simulink model "case8"  (R2024b)
settings: Solver=FixedStepAuto  StartTime=0  StopTime=1  FixedStep=1e-7  RelTol=1e-3
values from neighbouring files (symbols this model uses):
  SG_D_1_D = 0.01056    [IEEE9_case_parameters.m]    (also in case1_parameters.m; case2_parameters.m; case3_parameters.m; case4_parameters.m)
  SG_D_1_EnableSaturation = 0    [IEEE9_case_parameters.m]    (also in case1_parameters.m; case2_parameters.m; case3_parameters.m; case4_parameters.m)
  SG_D_1_f0 = 60    [IEEE9_case_parameters.m]    (also in case1_parameters.m; case2_parameters.m; case3_parameters.m; case4_parameters.m)
  SG_D_1_H = 7.5    [IEEE9_case_parameters.m]    (also in case1_parameters.m; case2_parameters.m; case3_parameters.m; case4_parameters.m)
  SG_D_1_K_A = 20    [IEEE9_case_parameters.m]    (also in case1_parameters.m; case2_parameters.m; case3_parameters.m; case4_parameters.m)
  SG_D_1_K_E = 1.000000e+1    (= 10)    [IEEE9_case_parameters.m]    (also in case1_parameters.m; case2_parameters.m; case3_parameters.m; case4_parameters.m)
  SG_D_1_K_F = 2.363    [IEEE9_case_parameters.m]    (also in case1_parameters.m; case2_parameters.m; case3_parameters.m; case4_parameters.m)
  SG_D_1_K_s = 0.5    [IEEE9_case_parameters.m]    (also in case1_parameters.m = 5; case2_parameters.m = 5; case3_parameters.m = 5; case4_parameters.m = 5)
  SG_D_1_R_a = 0.001088    [IEEE9_case_parameters.m]    (also in case1_parameters.m; case2_parameters.m; case3_parameters.m; case4_parameters.m)
  SG_D_1_S_A = 1    [IEEE9_case_parameters.m]    (also in case1_parameters.m; case2_parameters.m; case3_parameters.m; case4_parameters.m)
  SG_D_1_S_B = 0.103    [IEEE9_case_parameters.m]    (also in case1_parameters.m; case2_parameters.m; case3_parameters.m; case4_parameters.m)
  SG_D_1_S_N = 10.659857    [IEEE9_case_parameters.m]    (also in case1_parameters.m; case2_parameters.m; case3_parameters.m; case4_parameters.m)
  SG_D_1_SpeedPara = 200    [IEEE9_case_parameters.m]    (also in case1_parameters.m; case2_parameters.m; case3_parameters.m; case4_parameters.m)
  SG_D_1_T_0 = 0.720173    [IEEE9_case_parameters.m]    (also in case1_parameters.m = 0.755522; case2_parameters.m = 0.808931; case3_parameters.m = 0.869402; case4_parameters.m = 0.729316)
  SG_D_1_T_1 = 0.3    [IEEE9_case_parameters.m]    (also in case1_parameters.m; case2_parameters.m; case3_parameters.m; case4_parameters.m)
  SG_D_1_T_2 = 0.05    [IEEE9_case_parameters.m]    (also in case1_parameters.m; case2_parameters.m; case3_parameters.m; case4_parameters.m)
  SG_D_1_T_3 = 0.02    [IEEE9_case_parameters.m]    (also in case1_parameters.m; case2_parameters.m; case3_parameters.m; case4_parameters.m)
  SG_D_1_T_4 = 0.005    [IEEE9_case_parameters.m]    (also in case1_parameters.m; case2_parameters.m; case3_parameters.m; case4_parameters.m)
  SG_D_1_T_A = 0.02    [IEEE9_case_parameters.m]    (also in case1_parameters.m; case2_parameters.m; case3_parameters.m; case4_parameters.m)
  SG_D_1_T_dd = 8.000000e+0    (= 8)    [IEEE9_case_parameters.m]    (also in case1_parameters.m; case2_parameters.m; case3_parameters.m; case4_parameters.m)
  SG_D_1_T_ddd = 0.04    [IEEE9_case_parameters.m]    (also in case1_parameters.m; case2_parameters.m; case3_parameters.m; case4_parameters.m)
  SG_D_1_T_E = 0.314    [IEEE9_case_parameters.m]    (also in case1_parameters.m; case2_parameters.m; case3_parameters.m; case4_parameters.m)
  SG_D_1_T_F = 0.35    [IEEE9_case_parameters.m]    (also in case1_parameters.m; case2_parameters.m; case3_parameters.m; case4_parameters.m)
  SG_D_1_T_qd = 0.8    [IEEE9_case_parameters.m]    (also in case1_parameters.m; case2_parameters.m; case3_parameters.m; case4_parameters.m)
  SG_D_1_T_qdd = 0.02    [IEEE9_case_parameters.m]    (also in case1_parameters.m; case2_parameters.m; case3_parameters.m; case4_parameters.m)
  SG_D_1_T_speed = 0.1    [IEEE9_case_parameters.m]    (also in case1_parameters.m = 200; case2_parameters.m = 200; case3_parameters.m = 200; case4_parameters.m = 200)
  SG_D_1_T_w = 0.5    [IEEE9_case_parameters.m]    (also in case1_parameters.m; case2_parameters.m; case3_parameters.m; case4_parameters.m)
  SG_D_1_V_ref = 1.990276    [IEEE9_case_parameters.m]    (also in case1_parameters.m = 2.042296; case2_parameters.m = 2.051388; case3_parameters.m = 2.089584; case4_parameters.m = 2.01845)
  SG_D_1_w_ref = 376.991118    [IEEE9_case_parameters.m]    (also in case1_parameters.m; case2_parameters.m; case3_parameters.m; case4_parameters.m)
  SG_D_1_wb = 6.000000e+1    (= 60)    [IEEE9_case_parameters.m]    (also in case1_parameters.m; case2_parameters.m; case3_parameters.m; case4_parameters.m)
  SG_D_1_x_d = 1.9    [IEEE9_case_parameters.m]    (also in case1_parameters.m; case2_parameters.m; case3_parameters.m; case4_parameters.m)
  SG_D_1_x_dd = 0.302    [IEEE9_case_parameters.m]    (also in case1_parameters.m; case2_parameters.m; case3_parameters.m; case4_parameters.m)
  SG_D_1_x_ddd = 0.204    [IEEE9_case_parameters.m]    (also in case1_parameters.m; case2_parameters.m; case3_parameters.m; case4_parameters.m)
  SG_D_1_x_l = 0.05    [IEEE9_case_parameters.m]    (also in case1_parameters.m; case2_parameters.m; case3_parameters.m; case4_parameters.m)
  SG_D_1_x_q = 1.3    [IEEE9_case_parameters.m]    (also in case1_parameters.m; case2_parameters.m; case3_parameters.m; case4_parameters.m)
  SG_D_1_x_qd = 0.5    [IEEE9_case_parameters.m]    (also in case1_parameters.m; case2_parameters.m; case3_parameters.m; case4_parameters.m)
  SG_D_1_x_qdd = 0.3    [IEEE9_case_parameters.m]    (also in case1_parameters.m; case2_parameters.m; case3_parameters.m; case4_parameters.m)
  SG_D_2_D = 0.02    [IEEE9_case_parameters.m]    (also in case1_parameters.m; case2_parameters.m; case3_parameters.m; case4_parameters.m)
  SG_D_2_EnableSaturation = 0    [IEEE9_case_parameters.m]    (also in case1_parameters.m; case2_parameters.m; case3_parameters.m; case4_parameters.m)
  SG_D_2_f0 = 60    [IEEE9_case_parameters.m]    (also in case1_parameters.m; case2_parameters.m; case3_parameters.m; case4_parameters.m)
  SG_D_2_H = 8.000000e+0    (= 8)    [IEEE9_case_parameters.m]    (also in case1_parameters.m; case2_parameters.m; case3_parameters.m; case4_parameters.m)
  SG_D_2_K_A = 20    [IEEE9_case_parameters.m]    (also in case1_parameters.m; case2_parameters.m; case3_parameters.m; case4_parameters.m)
  SG_D_2_K_E = 1.000000e+1    (= 10)    [IEEE9_case_parameters.m]    (also in case1_parameters.m; case2_parameters.m; case3_parameters.m; case4_parameters.m)
  SG_D_2_K_F = 2.363    [IEEE9_case_parameters.m]    (also in case1_parameters.m; case2_parameters.m; case3_parameters.m; case4_parameters.m)
  SG_D_2_K_s = 0.5    [IEEE9_case_parameters.m]    (also in case1_parameters.m = 4; case2_parameters.m = 4; case3_parameters.m = 4; case4_parameters.m = 4)
  SG_D_2_R_a = 0.001088    [IEEE9_case_parameters.m]    (also in case1_parameters.m; case2_parameters.m; case3_parameters.m; case4_parameters.m)
  SG_D_2_S_A = 1    [IEEE9_case_parameters.m]    (also in case1_parameters.m; case2_parameters.m; case3_parameters.m; case4_parameters.m)
  SG_D_2_S_B = 0.103    [IEEE9_case_parameters.m]    (also in case1_parameters.m; case2_parameters.m; case3_parameters.m; case4_parameters.m)
  SG_D_2_S_N = 10.659857    [IEEE9_case_parameters.m]    (also in case1_parameters.m; case2_parameters.m; case3_parameters.m; case4_parameters.m)
  SG_D_2_SpeedPara = 200    [IEEE9_case_parameters.m]    (also in case1_parameters.m; case2_parameters.m; case3_parameters.m; case4_parameters.m)
  SG_D_2_T_0 = 1.632913    [IEEE9_case_parameters.m]    (also in case1_parameters.m = 1.632925; case2_parameters.m = 1.632915; case3_parameters.m = 1.632914; case4_parameters.m = 1.632927)
  SG_D_2_T_1 = 0.2    [IEEE9_case_parameters.m]    (also in case1_parameters.m; case2_parameters.m; case3_parameters.m; case4_parameters.m)
  SG_D_2_T_2 = 0.05    [IEEE9_case_parameters.m]    (also in case1_parameters.m; case2_parameters.m; case3_parameters.m; case4_parameters.m)
  SG_D_2_T_3 = 0.02    [IEEE9_case_parameters.m]    (also in case1_parameters.m; case2_parameters.m; case3_parameters.m; case4_parameters.m)
  SG_D_2_T_4 = 0.005    [IEEE9_case_parameters.m]    (also in case1_parameters.m; case2_parameters.m; case3_parameters.m; case4_parameters.m)
  SG_D_2_T_A = 0.02    [IEEE9_case_parameters.m]    (also in case1_parameters.m; case2_parameters.m; case3_parameters.m; case4_parameters.m)
  SG_D_2_T_dd = 7.9    [IEEE9_case_parameters.m]    (also in case1_parameters.m; case2_parameters.m; case3_parameters.m; case4_parameters.m)
  SG_D_2_T_ddd = 0.04    [IEEE9_case_parameters.m]    (also in case1_parameters.m; case2_parameters.m; case3_parameters.m; case4_parameters.m)
  SG_D_2_T_E = 0.314    [IEEE9_case_parameters.m]    (also in case1_parameters.m; case2_parameters.m; case3_parameters.m; case4_parameters.m)
  SG_D_2_T_F = 0.35    [IEEE9_case_parameters.m]    (also in case1_parameters.m; case2_parameters.m; case3_parameters.m; case4_parameters.m)
  SG_D_2_T_qd = 0.8    [IEEE9_case_parameters.m]    (also in case1_parameters.m; case2_parameters.m; case3_parameters.m; case4_parameters.m)
  SG_D_2_T_qdd = 0.015    [IEEE9_case_parameters.m]    (also in case1_parameters.m; case2_parameters.m; case3_parameters.m; case4_parameters.m)
  SG_D_2_T_speed = 0.1    [IEEE9_case_parameters.m]    (also in case1_parameters.m = 150; case2_parameters.m = 150; case3_parameters.m = 150; case4_parameters.m = 150)
  SG_D_2_T_w = 0.35    [IEEE9_case_parameters.m]    (also in case1_parameters.m; case2_parameters.m; case3_parameters.m; case4_parameters.m)
  SG_D_2_V_ref = 2.58547    [IEEE9_case_parameters.m]    (also in case1_parameters.m = 2.597896; case2_parameters.m = 2.587136; case3_parameters.m = 2.586042; case4_parameters.m = 2.599679)
  SG_D_2_w_ref = 376.991118    [IEEE9_case_parameters.m]    (also in case1_parameters.m; case2_parameters.m; case3_parameters.m; case4_parameters.m)
  SG_D_2_wb = 6.000000e+1    (= 60)    [IEEE9_case_parameters.m]    (also in case1_parameters.m; case2_parameters.m; case3_parameters.m; case4_parameters.m)
  SG_D_2_x_d = 1.8    [IEEE9_case_parameters.m]    (also in case1_parameters.m; case2_parameters.m; case3_parameters.m; case4_parameters.m)
  SG_D_2_x_dd = 0.302    [IEEE9_case_parameters.m]    (also in case1_parameters.m; case2_parameters.m; case3_parameters.m; case4_parameters.m)
  SG_D_2_x_ddd = 0.204    [IEEE9_case_parameters.m]    (also in case1_parameters.m; case2_parameters.m; case3_parameters.m; case4_parameters.m)
  SG_D_2_x_l = 0.05    [IEEE9_case_parameters.m]    (also in case1_parameters.m; case2_parameters.m; case3_parameters.m; case4_parameters.m)
  SG_D_2_x_q = 1.25    [IEEE9_case_parameters.m]    (also in case1_parameters.m; case2_parameters.m; case3_parameters.m; case4_parameters.m)
  SG_D_2_x_qd = 0.5    [IEEE9_case_parameters.m]    (also in case1_parameters.m; case2_parameters.m; case3_parameters.m; case4_parameters.m)
  SG_D_2_x_qdd = 0.3    [IEEE9_case_parameters.m]    (also in case1_parameters.m; case2_parameters.m; case3_parameters.m; case4_parameters.m)
  SG_D_3_D = 0.02    [IEEE9_case_parameters.m]    (also in case1_parameters.m; case2_parameters.m; case3_parameters.m; case4_parameters.m)
  SG_D_3_EnableSaturation = 0    [IEEE9_case_parameters.m]    (also in case1_parameters.m; case2_parameters.m; case3_parameters.m; case4_parameters.m)
  SG_D_3_f0 = 60    [IEEE9_case_parameters.m]    (also in case1_parameters.m; case2_parameters.m; case3_parameters.m; case4_parameters.m)
  SG_D_3_H = 7.7    [IEEE9_case_parameters.m]    (also in case1_parameters.m; case2_parameters.m; case3_parameters.m; case4_parameters.m)
  SG_D_3_K_A = 20    [IEEE9_case_parameters.m]    (also in case1_parameters.m; case2_parameters.m; case3_parameters.m; case4_parameters.m)
  SG_D_3_K_E = 1.000000e+1    (= 10)    [IEEE9_case_parameters.m]    (also in case1_parameters.m; case2_parameters.m; case3_parameters.m; case4_parameters.m)
  SG_D_3_K_F = 2.363    [IEEE9_case_parameters.m]    (also in case1_parameters.m; case2_parameters.m; case3_parameters.m; case4_parameters.m)
  SG_D_3_K_s = 0.2    [IEEE9_case_parameters.m]    (also in case1_parameters.m = 2; case2_parameters.m = 2; case3_parameters.m = 2; case4_parameters.m = 2)
  SG_D_3_R_a = 0.001088    [IEEE9_case_parameters.m]    (also in case1_parameters.m; case2_parameters.m; case3_parameters.m; case4_parameters.m)
  SG_D_3_S_A = 1    [IEEE9_case_parameters.m]    (also in case1_parameters.m; case2_parameters.m; case3_parameters.m; case4_parameters.m)
  SG_D_3_S_B = 0.103    [IEEE9_case_parameters.m]    (also in case1_parameters.m; case2_parameters.m; case3_parameters.m; case4_parameters.m)
  SG_D_3_S_N = 10.659857    [IEEE9_case_parameters.m]    (also in case1_parameters.m; case2_parameters.m; case3_parameters.m; case4_parameters.m)
  SG_D_3_SpeedPara = 200    [IEEE9_case_parameters.m]    (also in case1_parameters.m; case2_parameters.m; case3_parameters.m; case4_parameters.m)
  SG_D_3_T_0 = 0.850788    [IEEE9_case_parameters.m]    (also in case1_parameters.m = 0.850786; case2_parameters.m = 0.850787; case3_parameters.m; case4_parameters.m = 0.850786)
  SG_D_3_T_1 = 0.2    [IEEE9_case_parameters.m]    (also in case1_parameters.m; case2_parameters.m; case3_parameters.m; case4_parameters.m)
  SG_D_3_T_2 = 0.05    [IEEE9_case_parameters.m]    (also in case1_parameters.m; case2_parameters.m; case3_parameters.m; case4_parameters.m)
  SG_D_3_T_3 = 0.02    [IEEE9_case_parameters.m]    (also in case1_parameters.m; case2_parameters.m; case3_parameters.m; case4_parameters.m)
  SG_D_3_T_4 = 0.005    [IEEE9_case_parameters.m]    (also in case1_parameters.m; case2_parameters.m; case3_parameters.m; case4_parameters.m)
  SG_D_3_T_A = 0.02    [IEEE9_case_parameters.m]    (also in case1_parameters.m; case2_parameters.m; case3_parameters.m; case4_parameters.m)
  SG_D_3_T_dd = 8.1    [IEEE9_case_parameters.m]    (also in case1_parameters.m; case2_parameters.m; case3_parameters.m; case4_parameters.m)
  SG_D_3_T_ddd = 0.04    [IEEE9_case_parameters.m]    (also in case1_parameters.m; case2_parameters.m; case3_parameters.m; case4_parameters.m)
  SG_D_3_T_E = 0.314    [IEEE9_case_parameters.m]    (also in case1_parameters.m; case2_parameters.m; case3_parameters.m; case4_parameters.m)
  SG_D_3_T_F = 0.35    [IEEE9_case_parameters.m]    (also in case1_parameters.m; case2_parameters.m; case3_parameters.m; case4_parameters.m)
  SG_D_3_T_qd = 0.8    [IEEE9_case_parameters.m]    (also in case1_parameters.m; case2_parameters.m; case3_parameters.m; case4_parameters.m)
  SG_D_3_T_qdd = 0.015    [IEEE9_case_parameters.m]    (also in case1_parameters.m; case2_parameters.m; case3_parameters.m; case4_parameters.m)
  SG_D_3_T_speed = 0.1    [IEEE9_case_parameters.m]    (also in case1_parameters.m = 180; case2_parameters.m = 180; case3_parameters.m = 180; case4_parameters.m = 180)
  SG_D_3_T_w = 0.4    [IEEE9_case_parameters.m]    (also in case1_parameters.m; case2_parameters.m; case3_parameters.m; case4_parameters.m)
  SG_D_3_V_ref = 1.892727    [IEEE9_case_parameters.m]    (also in case1_parameters.m = 1.906439; case2_parameters.m = 1.895535; case3_parameters.m = 1.892105; case4_parameters.m = 1.906598)
  SG_D_3_w_ref = 376.991118    [IEEE9_case_parameters.m]    (also in case1_parameters.m; case2_parameters.m; case3_parameters.m; case4_parameters.m)
  SG_D_3_wb = 6.000000e+1    (= 60)    [IEEE9_case_parameters.m]    (also in case1_parameters.m; case2_parameters.m; case3_parameters.m; case4_parameters.m)
  SG_D_3_x_d = 1.85    [IEEE9_case_parameters.m]    (also in case1_parameters.m; case2_parameters.m; case3_parameters.m; case4_parameters.m)
  SG_D_3_x_dd = 0.302    [IEEE9_case_parameters.m]    (also in case1_parameters.m; case2_parameters.m; case3_parameters.m; case4_parameters.m)
  SG_D_3_x_ddd = 0.204    [IEEE9_case_parameters.m]    (also in case1_parameters.m; case2_parameters.m; case3_parameters.m; case4_parameters.m)
  SG_D_3_x_l = 0.05    [IEEE9_case_parameters.m]    (also in case1_parameters.m; case2_parameters.m; case3_parameters.m; case4_parameters.m)
  SG_D_3_x_q = 1.2    [IEEE9_case_parameters.m]    (also in case1_parameters.m; case2_parameters.m; case3_parameters.m; case4_parameters.m)
  SG_D_3_x_qd = 0.5    [IEEE9_case_parameters.m]    (also in case1_parameters.m; case2_parameters.m; case3_parameters.m; case4_parameters.m)
  SG_D_3_x_qdd = 0.3    [IEEE9_case_parameters.m]    (also in case1_parameters.m; case2_parameters.m; case3_parameters.m; case4_parameters.m)
(part 9 of 12)

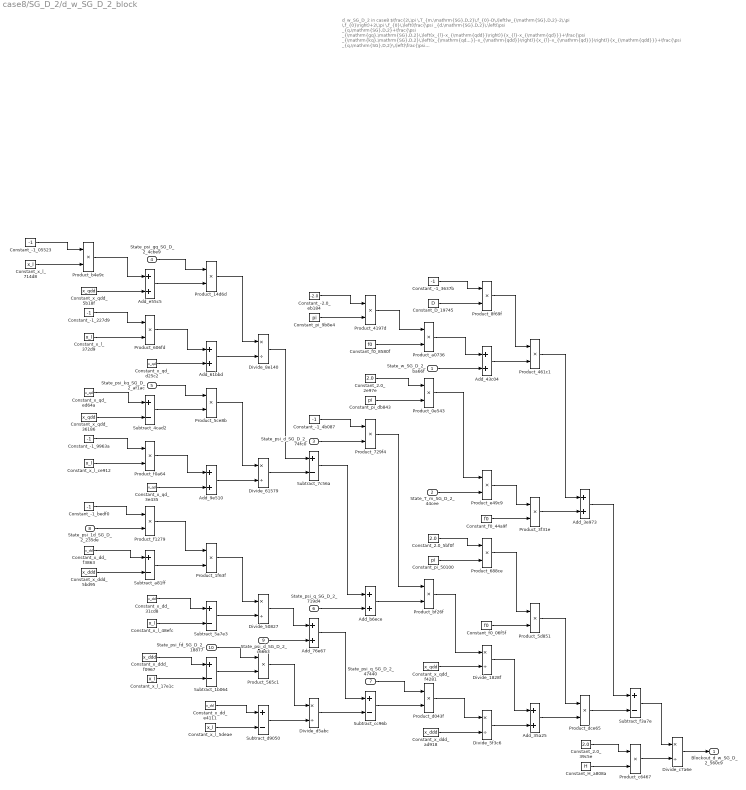
== system case8/SG_D_2/d_w_SG_D_2_block ==
  note: d_w_SG_D_2 in case8
      | $\frac{2\,\pi \,T_{m,\mathrm{SG},D,2}\,f_{0}-D\,\left(w_{\mathrm{SG},D,2}-2\,\pi \,f_{0}\right)+2\,\pi \,f_{0}\,\left(\frac{\psi _{d,\mathrm{SG},D,2}\,\left(\psi _{q,\mathrm{SG},D,2}+\frac{\psi _{\mathrm{gq},\mathrm{SG},D,2}\,\left(x_{l}-x_{\mathrm{qdd}}\right)}{x_{l}-x_{\mathrm{qd}}}+\frac{\psi _{\mathrm{kq},\mathrm{SG},D,2}\,\left(x_{\mathrm{qd}}-x_{\mathrm{qdd}}\right)}{x_{l}-x_{\mathrm{qd}}}\right)}{x_{\mathrm{qdd}}}+\frac{\psi _{q,\mathrm{SG},D,2}\,\left(\frac{\psi _{\mathrm{1d},\mathrm{SG},D,2}\,\left(x_{\mathrm{dd}}-x_{\mathrm{ddd}}\right)}{x_{\mathrm{dd}}-x_{l}}-\psi _{d,\mathrm{SG},D,2}+\frac{\psi _{\mathrm{fd},\mathrm{SG},D,2}\,\left(x_{\mathrm{ddd}}-x_{l}\right)}{x_{\mathrm{dd}}-x_{l}}\right)}{x_{\mathrm{ddd}}}\right)}{2\,H}$
      | Automatically generated on 2025-10-31 19:29:53 .
  State_w_SG_D_2_ba66f : Inport
  State_T_m_SG_D_2_44cee : Inport  Port=2
  State_psi_d_SG_D_2_74fc0 : Inport  Port=3
  State_psi_gq_SG_D_2_4cbe9 : Inport  Port=4
  State_psi_kq_SG_D_2_af1ac : Inport  Port=5
  State_psi_q_SG_D_2_719d4 : Inport  Port=6
  State_psi_q_SG_D_2_47440 : Inport  Port=7
  State_psi_1d_SG_D_2_235de : Inport  Port=8
  State_psi_d_SG_D_2_c6663 : Inport  Port=9
  State_psi_fd_SG_D_2_18877 : Inport  Port=10
  Add_35a25 : Sum
  Add_3e973 : Sum
  Add_43c04 : Sum
  Add_61bbd : Sum
  Add_76e67 : Sum
  Add_9e510 : Sum
  Add_b6ece : Sum
  Add_e55c5 : Sum
  Constant_-1_05523 : Constant  Value=-1
  Constant_-1_227d9 : Constant  Value=-1
  Constant_-1_3637b : Constant  Value=-1
  Constant_-1_4b087 : Constant  Value=-1
  Constant_-1_9963a : Constant  Value=-1
  Constant_-1_bedf0 : Constant  Value=-1
  Constant_-2.0_eb184 : Constant  Value=-2.0
  Constant_2.0_2e97e : Constant  Value=2.0
  Constant_2.0_39c5e : Constant  Value=2.0
  Constant_2.0_5bf0f : Constant  Value=2.0
  Constant_D_19745 : Constant  Value=D
  Constant_H_a808a : Constant  Value=H
  Constant_f0_06f5f : Constant  Value=f0
  Constant_f0_44a9f : Constant  Value=f0
  Constant_f0_8580f : Constant  Value=f0
  Constant_pi_50100 : Constant  Value=pi
  Constant_pi_9b8e4 : Constant  Value=pi
  Constant_pi_db843 : Constant  Value=pi
  Constant_x_dd_31cd8 : Constant  Value=x_dd
  Constant_x_dd_e4111 : Constant  Value=x_dd
  Constant_x_dd_f3863 : Constant  Value=x_dd
  Constant_x_ddd_5bd95 : Constant  Value=x_ddd
  Constant_x_ddd_ad918 : Constant  Value=x_ddd
  Constant_x_ddd_f0967 : Constant  Value=x_ddd
  Constant_x_l_17e1c : Constant  Value=x_l
  Constant_x_l_372d9 : Constant  Value=x_l
  Constant_x_l_48efc : Constant  Value=x_l
  Constant_x_l_5deae : Constant  Value=x_l
  Constant_x_l_714d8 : Constant  Value=x_l
  Constant_x_l_ce912 : Constant  Value=x_l
  Constant_x_qd_3e435 : Constant  Value=x_qd
  Constant_x_qd_d25c2 : Constant  Value=x_qd
  Constant_x_qd_ed64a : Constant  Value=x_qd
  Constant_x_qdd_36186 : Constant  Value=x_qdd
  Constant_x_qdd_5b18f : Constant  Value=x_qdd
  Constant_x_qdd_f4281 : Constant  Value=x_qdd
  Divide_1828f : Product  Inputs=*/
  Divide_50827 : Product  Inputs=*/
  Divide_5f3c6 : Product  Inputs=*/
  Divide_61579 : Product  Inputs=*/
  Divide_8e140 : Product  Inputs=*/
  Divide_c7a6e : Product  Inputs=*/
  Divide_d5abc : Product  Inputs=*/
  Product_0e543 : Product
  Product_14d6d : Product
  Product_1f63f : Product
  Product_3f31e : Product
  Product_4197d : Product
  Product_461c1 : Product
  Product_565c1 : Product
  Product_5ce8b : Product
  Product_5d851 : Product
  Product_606fd : Product
  Product_688ce : Product
  Product_729f4 : Product
  Product_8f69f : Product
  Product_a0736 : Product
  Product_b4e9c : Product
  Product_bf26f : Product
  Product_c6467 : Product
  Product_d043f : Product
  Product_dce65 : Product
  Product_e49c9 : Product
  Product_f0a64 : Product
  Product_f1279 : Product
  Subtract_1b064 : Sum  Inputs=+-
  Subtract_4cad2 : Sum  Inputs=+-
  Subtract_5a7e3 : Sum  Inputs=+-
  Subtract_7c56a : Sum  Inputs=+-
  Subtract_a81ff : Sum  Inputs=+-
  Subtract_cc96b : Sum  Inputs=+-
  Subtract_d9050 : Sum  Inputs=+-
  Subtract_f3a7e : Sum  Inputs=+-
  Blockout_d_w_SG_D_2_560c9 : Outport
  wires:
  Constant_x_qd_ed64a/1 -> Subtract_4cad2/1
  Constant_-1_9963a/1 -> Product_f0a64/1
  Constant_-1_05523/1 -> Product_b4e9c/1
  Constant_x_qdd_36186/1 -> Subtract_4cad2/2
  Subtract_d9050/1 -> Divide_d5abc/2
  Constant_x_l_ce912/1 -> Product_f0a64/2
  Constant_x_l_714d8/1 -> Product_b4e9c/2
  Product_f0a64/1 -> Add_9e510/1
  Product_b4e9c/1 -> Add_e55c5/1
  Constant_x_l_48efc/1 -> Subtract_5a7e3/2
  Constant_x_l_372d9/1 -> Product_606fd/2
  Constant_x_ddd_ad918/1 -> Divide_5f3c6/2
  Subtract_1b064/1 -> Product_565c1/2
  Constant_x_qd_3e435/1 -> Add_9e510/2
  Constant_x_qdd_5b18f/1 -> Add_e55c5/2
  Constant_-1_227d9/1 -> Product_606fd/1
  State_psi_d_SG_D_2_74fc0/1 -> Product_729f4/2
  Constant_-1_bedf0/1 -> Product_f1279/1
  State_w_SG_D_2_ba66f/1 -> Add_43c04/2
  Product_606fd/1 -> Add_61bbd/1
  State_psi_1d_SG_D_2_235de/1 -> Product_f1279/2
  Constant_x_dd_f3863/1 -> Subtract_a81ff/1
  Divide_8e140/1 -> Subtract_7c56a/1
  Subtract_4cad2/1 -> Product_5ce8b/2
  Constant_x_ddd_5bd95/1 -> Subtract_a81ff/2
  State_psi_gq_SG_D_2_4cbe9/1 -> Product_14d6d/1
  Add_9e510/1 -> Divide_61579/2
  State_psi_d_SG_D_2_c6663/1 -> Add_76e67/2
  Add_e55c5/1 -> Product_14d6d/2
  Constant_x_qd_d25c2/1 -> Add_61bbd/2
  State_psi_kq_SG_D_2_af1ac/1 -> Product_5ce8b/1
  Product_f1279/1 -> Product_1f63f/1
  Subtract_a81ff/1 -> Product_1f63f/2
  Constant_pi_db843/1 -> Product_0e543/2
  Constant_x_dd_31cd8/1 -> Subtract_5a7e3/1
  Constant_x_ddd_f0967/1 -> Subtract_1b064/1
  Constant_x_l_17e1c/1 -> Subtract_1b064/2
  Product_14d6d/1 -> Divide_8e140/1
  Add_61bbd/1 -> Divide_8e140/2
  Add_b6ece/1 -> Product_bf26f/2
  Product_5ce8b/1 -> Divide_61579/1
  Constant_pi_9b8e4/1 -> Product_4197d/2
  Product_1f63f/1 -> Divide_50827/1
  Subtract_5a7e3/1 -> Divide_50827/2
  State_psi_fd_SG_D_2_18877/1 -> Product_565c1/1
  Divide_50827/1 -> Add_76e67/1
  Constant_x_dd_e4111/1 -> Subtract_d9050/1
  Constant_x_l_5deae/1 -> Subtract_d9050/2
  Divide_61579/1 -> Subtract_7c56a/2
  Product_565c1/1 -> Divide_d5abc/1
  Constant_-1_4b087/1 -> Product_729f4/1
  Constant_-2.0_eb184/1 -> Product_4197d/1
  Subtract_7c56a/1 -> Add_b6ece/1
  Subtract_cc96b/1 -> Product_d043f/2
  State_psi_q_SG_D_2_719d4/1 -> Add_b6ece/2
  Constant_D_19745/1 -> Product_8f69f/2
  Add_76e67/1 -> Subtract_cc96b/1
  Divide_d5abc/1 -> Subtract_cc96b/2
  Product_4197d/1 -> Product_a0736/1
  Constant_f0_8580f/1 -> Product_a0736/2
  Constant_2.0_2e97e/1 -> Product_0e543/1
  Product_729f4/1 -> Product_bf26f/1
  State_psi_q_SG_D_2_47440/1 -> Product_d043f/1
  Constant_-1_3637b/1 -> Product_8f69f/1
  Product_a0736/1 -> Add_43c04/1
  Product_0e543/1 -> Product_e49c9/1
  State_T_m_SG_D_2_44cee/1 -> Product_e49c9/2
  Constant_2.0_5bf0f/1 -> Product_688ce/1
  Constant_pi_50100/1 -> Product_688ce/2
  Product_bf26f/1 -> Divide_1828f/1
  Constant_x_qdd_f4281/1 -> Divide_1828f/2
  Product_d043f/1 -> Divide_5f3c6/1
  Product_8f69f/1 -> Product_461c1/1
  Add_43c04/1 -> Product_461c1/2
  Product_e49c9/1 -> Product_3f31e/1
  Constant_f0_44a9f/1 -> Product_3f31e/2
  Product_688ce/1 -> Product_5d851/1
  Constant_f0_06f5f/1 -> Product_5d851/2
  Divide_1828f/1 -> Add_35a25/1
  Divide_5f3c6/1 -> Add_35a25/2
  Product_461c1/1 -> Add_3e973/1
  Product_3f31e/1 -> Add_3e973/2
  Product_5d851/1 -> Product_dce65/1
  Add_35a25/1 -> Product_dce65/2
  Add_3e973/1 -> Subtract_f3a7e/1
  Product_dce65/1 -> Subtract_f3a7e/2
  Constant_2.0_39c5e/1 -> Product_c6467/1
  Constant_H_a808a/1 -> Product_c6467/2
  Subtract_f3a7e/1 -> Divide_c7a6e/1
  Product_c6467/1 -> Divide_c7a6e/2
  Divide_c7a6e/1 -> Blockout_d_w_SG_D_2_560c9/1

== system case8/SG_D_2/i_d_SG_D_2_block ==
  note: i_d_SG_D_2 in case8
      | $\frac{\sin\left(\theta _{\mathrm{SG},D,2}\right)\,\left(\frac{\psi _{\mathrm{1d},\mathrm{SG},D,2}\,\left(x_{\mathrm{dd}}-x_{\mathrm{ddd}}\right)}{x_{\mathrm{dd}}-x_{l}}-\psi _{d,\mathrm{SG},D,2}+\frac{\psi _{\mathrm{fd},\mathrm{SG},D,2}\,\left(x_{\mathrm{ddd}}-x_{l}\right)}{x_{\mathrm{dd}}-x_{l}}\right)}{x_{\mathrm{ddd}}}-\frac{\cos\left(\theta _{\mathrm{SG},D,2}\right)\,\left(\psi _{q,\mathrm{SG},D,2}+\frac{\psi _{\mathrm{gq},\mathrm{SG},D,2}\,\left(x_{l}-x_{\mathrm{qdd}}\right)}{x_{l}-x_{\mathrm{qd}}}+\frac{\psi _{\mathrm{kq},\mathrm{SG},D,2}\,\left(x_{\mathrm{qd}}-x_{\mathrm{qdd}}\right)}{x_{l}-x_{\mathrm{qd}}}\right)}{x_{\mathrm{qdd}}}$
      | Automatically generated on 2025-10-31 19:29:59 .
  State_psi_gq_SG_D_2_6632a : Inport
  State_psi_kq_SG_D_2_999f9 : Inport  Port=2
  State_psi_q_SG_D_2_62810 : Inport  Port=3
  State_theta_SG_D_2_8321e : Inport  Port=4
  State_psi_1d_SG_D_2_4ff2d : Inport  Port=5
  State_psi_d_SG_D_2_05ecc : Inport  Port=6
  State_psi_fd_SG_D_2_bfe7a : Inport  Port=7
  State_theta_SG_D_2_8d67b : Inport  Port=8
  Add_20ed7 : Sum
  Add_3dc6c : Sum
  Add_5c646 : Sum
  Add_7b709 : Sum
  Add_e6514 : Sum
  Constant_-1_3d246 : Constant  Value=-1
  Constant_-1_3feff : Constant  Value=-1
  Constant_-1_414e4 : Constant  Value=-1
  Constant_-1_75017 : Constant  Value=-1
  Constant_-1_ee62c : Constant  Value=-1
  Constant_x_dd_6341c : Constant  Value=x_dd
  Constant_x_dd_aa2bd : Constant  Value=x_dd
  Constant_x_dd_bd271 : Constant  Value=x_dd
  Constant_x_ddd_37e59 : Constant  Value=x_ddd
  Constant_x_ddd_8b57c : Constant  Value=x_ddd
  Constant_x_ddd_99cdf : Constant  Value=x_ddd
  Constant_x_l_57dce : Constant  Value=x_l
  Constant_x_l_63788 : Constant  Value=x_l
  Constant_x_l_78c75 : Constant  Value=x_l
  Constant_x_l_9be85 : Constant  Value=x_l
  Constant_x_l_be7fe : Constant  Value=x_l
  Constant_x_l_ed492 : Constant  Value=x_l
  Constant_x_qd_4982c : Constant  Value=x_qd
  Constant_x_qd_6d963 : Constant  Value=x_qd
  Constant_x_qd_fe70c : Constant  Value=x_qd
  Constant_x_qdd_70aeb : Constant  Value=x_qdd
  Constant_x_qdd_ca87c : Constant  Value=x_qdd
  Constant_x_qdd_ed072 : Constant  Value=x_qdd
  Divide_2e497 : Product  Inputs=*/
  Divide_6b875 : Product  Inputs=*/
  Divide_9db00 : Product  Inputs=*/
  Divide_a4e61 : Product  Inputs=*/
  Divide_a6fb4 : Product  Inputs=*/
  Divide_cb703 : Product  Inputs=*/
  MathFunc_cos_48262 : Trigonometry  Operator=cos
  MathFunc_sin_7da68 : Trigonometry
  Product_3fa10 : Product
  Product_5b25c : Product
  Product_714a4 : Product
  Product_81a9f : Product
  Product_91ddb : Product
  Product_9e80c : Product
  Product_b7a82 : Product
  Product_c45a5 : Product
  Product_d08c5 : Product
  Product_daef6 : Product
  Product_e15e2 : Product
  Subtract_13aa5 : Sum  Inputs=+-
  Subtract_45d0b : Sum  Inputs=+-
  Subtract_4b65b : Sum  Inputs=+-
  Subtract_561b3 : Sum  Inputs=+-
  Subtract_58675 : Sum  Inputs=+-
  Subtract_de34d : Sum  Inputs=+-
  Subtract_e4056 : Sum  Inputs=+-
  Subtract_e8187 : Sum  Inputs=+-
  Blockout_i_d_SG_D_2_06834 : Outport
  wires:
  Constant_x_ddd_99cdf/1 -> Subtract_e8187/1
  Constant_x_qd_4982c/1 -> Subtract_4b65b/1
  Constant_-1_3d246/1 -> Product_3fa10/1
  Constant_-1_ee62c/1 -> Product_c45a5/1
  Subtract_13aa5/1 -> Blockout_i_d_SG_D_2_06834/1
  Constant_x_qdd_ed072/1 -> Subtract_4b65b/2
  Constant_x_l_57dce/1 -> Product_3fa10/2
  Constant_x_l_9be85/1 -> Product_c45a5/2
  Product_3fa10/1 -> Add_e6514/1
  Product_c45a5/1 -> Add_5c646/1
  Constant_x_l_be7fe/1 -> Product_81a9f/2
  Constant_x_qd_6d963/1 -> Add_e6514/2
  Constant_x_qdd_70aeb/1 -> Add_5c646/2
  Constant_x_qdd_ca87c/1 -> Divide_9db00/2
  MathFunc_cos_48262/1 -> Product_714a4/2
  Constant_-1_3feff/1 -> Product_81a9f/1
  State_psi_gq_SG_D_2_6632a/1 -> Product_9e80c/1
  Subtract_e8187/1 -> Product_daef6/2
  Product_b7a82/1 -> Product_5b25c/1
  Add_e6514/1 -> Divide_a6fb4/2
  Add_5c646/1 -> Product_9e80c/2
  Product_daef6/1 -> Divide_6b875/1
  Product_81a9f/1 -> Add_7b709/1
  Constant_x_qd_fe70c/1 -> Add_7b709/2
  State_theta_SG_D_2_8d67b/1 -> MathFunc_sin_7da68/1
  State_psi_kq_SG_D_2_999f9/1 -> Product_e15e2/1
  Add_3dc6c/1 -> Subtract_561b3/1
  Subtract_4b65b/1 -> Product_e15e2/2
  Product_9e80c/1 -> Divide_2e497/1
  Constant_-1_414e4/1 -> Product_b7a82/1
  State_psi_1d_SG_D_2_4ff2d/1 -> Product_b7a82/2
  State_psi_fd_SG_D_2_bfe7a/1 -> Product_daef6/1
  Constant_x_dd_6341c/1 -> Subtract_45d0b/1
  Product_5b25c/1 -> Divide_cb703/1
  Constant_x_ddd_8b57c/1 -> Subtract_45d0b/2
  Divide_6b875/1 -> Subtract_561b3/2
  Add_7b709/1 -> Divide_2e497/2
  Product_d08c5/1 -> Divide_a4e61/1
  Product_e15e2/1 -> Divide_a6fb4/1
  Constant_-1_75017/1 -> Product_91ddb/1
  Subtract_de34d/1 -> Divide_6b875/2
  Subtract_45d0b/1 -> Product_5b25c/2
  Constant_x_dd_bd271/1 -> Subtract_e4056/1
  Subtract_561b3/1 -> Product_d08c5/1
  Constant_x_l_63788/1 -> Subtract_e4056/2
  Constant_x_l_78c75/1 -> Subtract_e8187/2
  Divide_2e497/1 -> Subtract_58675/1
  Divide_a4e61/1 -> Subtract_13aa5/2
  Divide_a6fb4/1 -> Subtract_58675/2
  Subtract_e4056/1 -> Divide_cb703/2
  Constant_x_dd_aa2bd/1 -> Subtract_de34d/1
  Divide_9db00/1 -> Subtract_13aa5/1
  Constant_x_l_ed492/1 -> Subtract_de34d/2
  Subtract_58675/1 -> Add_20ed7/1
  State_psi_q_SG_D_2_62810/1 -> Add_20ed7/2
  Constant_x_ddd_37e59/1 -> Divide_a4e61/2
  MathFunc_sin_7da68/1 -> Product_d08c5/2
  Divide_cb703/1 -> Add_3dc6c/1
  State_psi_d_SG_D_2_05ecc/1 -> Add_3dc6c/2
  Add_20ed7/1 -> Product_91ddb/2
  State_theta_SG_D_2_8321e/1 -> MathFunc_cos_48262/1
  Product_91ddb/1 -> Product_714a4/1
  Product_714a4/1 -> Divide_9db00/1

== system case8/SG_D_2/i_q_SG_D_2_block ==
  note: i_q_SG_D_2 in case8
      | $-\frac{\sin\left(\theta _{\mathrm{SG},D,2}\right)\,\left(\psi _{q,\mathrm{SG},D,2}+\frac{\psi _{\mathrm{gq},\mathrm{SG},D,2}\,\left(x_{l}-x_{\mathrm{qdd}}\right)}{x_{l}-x_{\mathrm{qd}}}+\frac{\psi _{\mathrm{kq},\mathrm{SG},D,2}\,\left(x_{\mathrm{qd}}-x_{\mathrm{qdd}}\right)}{x_{l}-x_{\mathrm{qd}}}\right)}{x_{\mathrm{qdd}}}-\frac{\cos\left(\theta _{\mathrm{SG},D,2}\right)\,\left(\frac{\psi _{\mathrm{1d},\mathrm{SG},D,2}\,\left(x_{\mathrm{dd}}-x_{\mathrm{ddd}}\right)}{x_{\mathrm{dd}}-x_{l}}-\psi _{d,\mathrm{SG},D,2}+\frac{\psi _{\mathrm{fd},\mathrm{SG},D,2}\,\left(x_{\mathrm{ddd}}-x_{l}\right)}{x_{\mathrm{dd}}-x_{l}}\right)}{x_{\mathrm{ddd}}}$
      | Automatically generated on 2025-10-31 19:30:00 .
  State_psi_gq_SG_D_2_ca4a4 : Inport
  State_psi_kq_SG_D_2_2a403 : Inport  Port=2
  State_psi_q_SG_D_2_6a090 : Inport  Port=3
  State_theta_SG_D_2_61b92 : Inport  Port=4
  State_psi_1d_SG_D_2_1de77 : Inport  Port=5
  State_psi_d_SG_D_2_04a53 : Inport  Port=6
  State_psi_fd_SG_D_2_88a91 : Inport  Port=7
  State_theta_SG_D_2_36c34 : Inport  Port=8
  Add_18fd8 : Sum
  Add_433fa : Sum
  Add_44b0b : Sum
  Add_688be : Sum
  Add_b4306 : Sum
  Add_b47f8 : Sum
  Constant_-1_7fe74 : Constant  Value=-1
  Constant_-1_88237 : Constant  Value=-1
  Constant_-1_a4e63 : Constant  Value=-1
  Constant_-1_db1f5 : Constant  Value=-1
  Constant_-1_f3200 : Constant  Value=-1
  Constant_x_dd_bfd44 : Constant  Value=x_dd
  Constant_x_dd_c0256 : Constant  Value=x_dd
  Constant_x_dd_e0c7a : Constant  Value=x_dd
  Constant_x_ddd_3cdad : Constant  Value=x_ddd
  Constant_x_ddd_85c6a : Constant  Value=x_ddd
  Constant_x_ddd_b6727 : Constant  Value=x_ddd
  Constant_x_l_0f6aa : Constant  Value=x_l
  Constant_x_l_3daef : Constant  Value=x_l
  Constant_x_l_68f53 : Constant  Value=x_l
  Constant_x_l_bf0ac : Constant  Value=x_l
  Constant_x_l_e2b88 : Constant  Value=x_l
  Constant_x_l_eec05 : Constant  Value=x_l
  Constant_x_qd_164d4 : Constant  Value=x_qd
  Constant_x_qd_b2471 : Constant  Value=x_qd
  Constant_x_qd_fa389 : Constant  Value=x_qd
  Constant_x_qdd_0f0f1 : Constant  Value=x_qdd
  Constant_x_qdd_3954d : Constant  Value=x_qdd
  Constant_x_qdd_da271 : Constant  Value=x_qdd
  Divide_04a2d : Product  Inputs=*/
  Divide_0bea4 : Product  Inputs=*/
  Divide_2bbdb : Product  Inputs=*/
  Divide_a094e : Product  Inputs=*/
  Divide_ce7c9 : Product  Inputs=*/
  Divide_d2f36 : Product  Inputs=*/
  MathFunc_cos_a469f : Trigonometry  Operator=cos
  MathFunc_sin_dd07b : Trigonometry
  Product_043f9 : Product
  Product_08070 : Product
  Product_08b78 : Product
  Product_27571 : Product
  Product_2fdc5 : Product
  Product_5a4ea : Product
  Product_7bc7c : Product
  Product_95f91 : Product
  Product_9aa63 : Product
  Product_a9bfd : Product
  Product_ebe48 : Product
  Subtract_0023b : Sum  Inputs=+-
  Subtract_46e79 : Sum  Inputs=+-
  Subtract_7393f : Sum  Inputs=+-
  Subtract_7beba : Sum  Inputs=+-
  Subtract_9eca7 : Sum  Inputs=+-
  Subtract_bd413 : Sum  Inputs=+-
  Subtract_e6b25 : Sum  Inputs=+-
  Blockout_i_q_SG_D_2_51e7b : Outport
  wires:
  MathFunc_sin_dd07b/1 -> Product_2fdc5/2
  Product_27571/1 -> Product_2fdc5/1
  Constant_-1_a4e63/1 -> Product_95f91/1
  Constant_-1_f3200/1 -> Product_9aa63/1
  Constant_x_l_eec05/1 -> Product_95f91/2
  Product_95f91/1 -> Add_44b0b/1
  Subtract_bd413/1 -> Product_08b78/2
  Constant_x_qdd_da271/1 -> Subtract_0023b/2
  Constant_x_qdd_0f0f1/1 -> Add_44b0b/2
  Add_433fa/1 -> Product_27571/2
  Constant_x_l_e2b88/1 -> Product_9aa63/2
  Constant_x_qd_164d4/1 -> Subtract_0023b/1
  Constant_-1_88237/1 -> Product_ebe48/1
  Constant_x_l_bf0ac/1 -> Product_ebe48/2
  State_psi_1d_SG_D_2_1de77/1 -> Product_7bc7c/2
  State_psi_gq_SG_D_2_ca4a4/1 -> Product_08070/1
  Add_44b0b/1 -> Product_08070/2
  Product_9aa63/1 -> Add_b4306/1
  Divide_a094e/1 -> Add_688be/1
  Constant_x_qd_fa389/1 -> Add_b4306/2
  State_psi_kq_SG_D_2_2a403/1 -> Product_5a4ea/1
  Add_b47f8/1 -> Subtract_7beba/1
  Constant_x_ddd_b6727/1 -> Subtract_bd413/2
  Subtract_0023b/1 -> Product_5a4ea/2
  Product_ebe48/1 -> Add_18fd8/1
  Constant_x_qd_b2471/1 -> Add_18fd8/2
  Constant_-1_7fe74/1 -> Product_7bc7c/1
  Constant_x_l_0f6aa/1 -> Subtract_7393f/2
  Constant_x_dd_c0256/1 -> Subtract_bd413/1
  Product_08070/1 -> Divide_0bea4/1
  Divide_d2f36/1 -> Subtract_7beba/2
  Add_b4306/1 -> Divide_0bea4/2
  Product_043f9/1 -> Divide_2bbdb/1
  Product_5a4ea/1 -> Divide_ce7c9/1
  Constant_-1_db1f5/1 -> Product_27571/1
  Product_7bc7c/1 -> Product_08b78/1
  Add_18fd8/1 -> Divide_ce7c9/2
  Constant_x_dd_e0c7a/1 -> Subtract_46e79/1
  Subtract_7beba/1 -> Product_043f9/1
  Subtract_e6b25/1 -> Product_a9bfd/2
  Constant_x_l_3daef/1 -> Subtract_46e79/2
  Constant_x_ddd_3cdad/1 -> Subtract_e6b25/1
  Constant_x_l_68f53/1 -> Subtract_e6b25/2
  Divide_0bea4/1 -> Subtract_9eca7/1
  Divide_2bbdb/1 -> Add_688be/2
  Product_a9bfd/1 -> Divide_d2f36/1
  Divide_ce7c9/1 -> Subtract_9eca7/2
  Subtract_7393f/1 -> Divide_d2f36/2
  Product_08b78/1 -> Divide_04a2d/1
  Subtract_46e79/1 -> Divide_04a2d/2
  Constant_x_qdd_3954d/1 -> Divide_a094e/2
  State_psi_fd_SG_D_2_88a91/1 -> Product_a9bfd/1
  Constant_x_dd_bfd44/1 -> Subtract_7393f/1
  Subtract_9eca7/1 -> Add_433fa/1
  State_psi_q_SG_D_2_6a090/1 -> Add_433fa/2
  Constant_x_ddd_85c6a/1 -> Divide_2bbdb/2
  Divide_04a2d/1 -> Add_b47f8/1
  State_psi_d_SG_D_2_04a53/1 -> Add_b47f8/2
  State_theta_SG_D_2_61b92/1 -> MathFunc_sin_dd07b/1
  State_theta_SG_D_2_36c34/1 -> MathFunc_cos_a469f/1
  MathFunc_cos_a469f/1 -> Product_043f9/2
  Product_2fdc5/1 -> Divide_a094e/1
  Add_688be/1 -> Blockout_i_q_SG_D_2_51e7b/1

== system case8/SG_D_2/theta_SG_D_2_out_block ==
  note: theta_SG_D_2_out in case8
      | $\theta _{\mathrm{SG},D,2}$
      | Automatically generated on 2025-10-31 19:30:02 .
  State_theta_SG_D_2_588b5 : Inport
  Blockout_theta_SG_D_2_out_80a64 : Outport
  wires:
  State_theta_SG_D_2_588b5/1 -> Blockout_theta_SG_D_2_out_80a64/1

== system case8/SG_D_2/w_SG_D_2_out_block ==
  note: w_SG_D_2_out in case8
      | $w_{\mathrm{SG},D,2}$
      | Automatically generated on 2025-10-31 19:30:01 .
  State_w_SG_D_2_c1838 : Inport
  Blockout_w_SG_D_2_out_5dbba : Outport
  wires:
  State_w_SG_D_2_c1838/1 -> Blockout_w_SG_D_2_out_5dbba/1

== system case8/SG_D_3/T_e_SG_D_3_block ==
  note: T_e_SG_D_3 in case8
      | $-\frac{\psi _{d,\mathrm{SG},D,3}\,\left(\psi _{q,\mathrm{SG},D,3}+\frac{\psi _{\mathrm{gq},\mathrm{SG},D,3}\,\left(x_{l}-x_{\mathrm{qdd}}\right)}{x_{l}-x_{\mathrm{qd}}}+\frac{\psi _{\mathrm{kq},\mathrm{SG},D,3}\,\left(x_{\mathrm{qd}}-x_{\mathrm{qdd}}\right)}{x_{l}-x_{\mathrm{qd}}}\right)}{x_{\mathrm{qdd}}}-\frac{\psi _{q,\mathrm{SG},D,3}\,\left(\frac{\psi _{\mathrm{1d},\mathrm{SG},D,3}\,\left(x_{\mathrm{dd}}-x_{\mathrm{ddd}}\right)}{x_{\mathrm{dd}}-x_{l}}-\psi _{d,\mathrm{SG},D,3}+\frac{\psi _{\mathrm{fd},\mathrm{SG},D,3}\,\left(x_{\mathrm{ddd}}-x_{l}\right)}{x_{\mathrm{dd}}-x_{l}}\right)}{x_{\mathrm{ddd}}}$
      | Automatically generated on 2025-10-31 19:30:20 .
  State_psi_d_SG_D_3_f2f0a : Inport
  State_psi_gq_SG_D_3_975c9 : Inport  Port=2
  State_psi_kq_SG_D_3_d23e5 : Inport  Port=3
  State_psi_q_SG_D_3_35d7e : Inport  Port=4
  State_psi_q_SG_D_3_c727a : Inport  Port=5
  State_psi_1d_SG_D_3_3c424 : Inport  Port=6
  State_psi_d_SG_D_3_7037a : Inport  Port=7
  State_psi_fd_SG_D_3_db5f7 : Inport  Port=8
  Add_0f2fe : Sum
  Add_37251 : Sum
  Add_450e1 : Sum
  Add_57115 : Sum
  Add_8033b : Sum
  Add_e4649 : Sum
  Constant_-1_46939 : Constant  Value=-1
  Constant_-1_5365c : Constant  Value=-1
  Constant_-1_605b0 : Constant  Value=-1
  Constant_-1_7356a : Constant  Value=-1
  Constant_-1_dfaa3 : Constant  Value=-1
  Constant_x_dd_3f50d : Constant  Value=x_dd
  Constant_x_dd_7b1d7 : Constant  Value=x_dd
  Constant_x_dd_c3f6e : Constant  Value=x_dd
  Constant_x_ddd_7e9fa : Constant  Value=x_ddd
  Constant_x_ddd_ead38 : Constant  Value=x_ddd
  Constant_x_ddd_f4348 : Constant  Value=x_ddd
  Constant_x_l_19c86 : Constant  Value=x_l
  Constant_x_l_288eb : Constant  Value=x_l
  Constant_x_l_36808 : Constant  Value=x_l
  Constant_x_l_7fb82 : Constant  Value=x_l
  Constant_x_l_9ecc1 : Constant  Value=x_l
  Constant_x_l_ac17a : Constant  Value=x_l
  Constant_x_qd_7740c : Constant  Value=x_qd
  Constant_x_qd_a5785 : Constant  Value=x_qd
  Constant_x_qd_e3e37 : Constant  Value=x_qd
  Constant_x_qdd_2ff73 : Constant  Value=x_qdd
  Constant_x_qdd_84d82 : Constant  Value=x_qdd
  Constant_x_qdd_f426e : Constant  Value=x_qdd
  Divide_6b655 : Product  Inputs=*/
  Divide_7c951 : Product  Inputs=*/
  Divide_b51b8 : Product  Inputs=*/
  Divide_ec37b : Product  Inputs=*/
  Divide_f995b : Product  Inputs=*/
  Divide_ff07e : Product  Inputs=*/
  Product_0ab9e : Product
  Product_1c4c8 : Product
  Product_2a4f7 : Product
  Product_3d604 : Product
  Product_3ebba : Product
  Product_419ad : Product
  Product_6d246 : Product
  Product_7aa92 : Product
  Product_aa6d6 : Product
  Product_b7b08 : Product
  Product_fb8e7 : Product
  Subtract_0c178 : Sum  Inputs=+-
  Subtract_49f1a : Sum  Inputs=+-
  Subtract_78436 : Sum  Inputs=+-
  Subtract_79cd2 : Sum  Inputs=+-
  Subtract_b5a37 : Sum  Inputs=+-
  Subtract_c35f8 : Sum  Inputs=+-
  Subtract_ec17f : Sum  Inputs=+-
  Blockout_T_e_SG_D_3_28e2c : Outport
  wires:
  State_psi_q_SG_D_3_35d7e/1 -> Add_57115/2
  Constant_-1_dfaa3/1 -> Product_3d604/1
  Subtract_ec17f/1 -> Product_419ad/2
  State_psi_1d_SG_D_3_3c424/1 -> Product_6d246/2
  Constant_-1_7356a/1 -> Product_0ab9e/1
  Constant_x_l_288eb/1 -> Product_0ab9e/2
  Add_450e1/1 -> Subtract_ec17f/1
  State_psi_d_SG_D_3_7037a/1 -> Add_450e1/2
  Product_0ab9e/1 -> Add_8033b/1
  Constant_x_qdd_f426e/1 -> Subtract_49f1a/2
  Add_57115/1 -> Product_7aa92/2
  Constant_x_qdd_84d82/1 -> Add_8033b/2
  State_psi_q_SG_D_3_c727a/1 -> Product_419ad/1
  Constant_x_l_36808/1 -> Product_3d604/2
  Subtract_78436/1 -> Divide_7c951/2
  Constant_x_l_19c86/1 -> Subtract_0c178/2
  Constant_x_qd_7740c/1 -> Subtract_49f1a/1
  Constant_-1_5365c/1 -> Product_b7b08/1
  Subtract_c35f8/1 -> Divide_b51b8/2
  Constant_x_l_ac17a/1 -> Product_b7b08/2
  Product_2a4f7/1 -> Divide_b51b8/1
  Constant_-1_605b0/1 -> Product_6d246/1
  Product_6d246/1 -> Product_2a4f7/1
  Constant_x_dd_c3f6e/1 -> Subtract_79cd2/1
  Constant_x_ddd_f4348/1 -> Subtract_79cd2/2
  Add_e4649/1 -> Blockout_T_e_SG_D_3_28e2c/1
  State_psi_gq_SG_D_3_975c9/1 -> Product_aa6d6/1
  Product_419ad/1 -> Divide_6b655/1
  Add_8033b/1 -> Product_aa6d6/2
  State_psi_fd_SG_D_3_db5f7/1 -> Product_fb8e7/1
  Product_3d604/1 -> Add_37251/1
  Constant_x_qd_e3e37/1 -> Add_37251/2
  Constant_x_dd_3f50d/1 -> Subtract_c35f8/1
  State_psi_kq_SG_D_3_d23e5/1 -> Product_1c4c8/1
  Constant_x_dd_7b1d7/1 -> Subtract_78436/1
  Subtract_49f1a/1 -> Product_1c4c8/2
  Product_7aa92/1 -> Divide_ff07e/1
  Product_b7b08/1 -> Add_0f2fe/1
  Add_37251/1 -> Divide_ec37b/2
  Constant_x_qd_a5785/1 -> Add_0f2fe/2
  Subtract_79cd2/1 -> Product_2a4f7/2
  Constant_x_l_7fb82/1 -> Subtract_c35f8/2
  Constant_x_ddd_ead38/1 -> Subtract_0c178/1
  Product_aa6d6/1 -> Divide_ec37b/1
  Product_1c4c8/1 -> Divide_f995b/1
  Add_0f2fe/1 -> Divide_f995b/2
  Constant_x_ddd_7e9fa/1 -> Divide_6b655/2
  Subtract_0c178/1 -> Product_fb8e7/2
  Divide_ec37b/1 -> Subtract_b5a37/1
  Constant_x_l_9ecc1/1 -> Subtract_78436/2
  Divide_f995b/1 -> Subtract_b5a37/2
  Divide_b51b8/1 -> Add_450e1/1
  Product_fb8e7/1 -> Divide_7c951/1
  Constant_-1_46939/1 -> Product_3ebba/1
  State_psi_d_SG_D_3_f2f0a/1 -> Product_3ebba/2
  Subtract_b5a37/1 -> Add_57115/1
  Divide_7c951/1 -> Subtract_ec17f/2
  Product_3ebba/1 -> Product_7aa92/1
  Constant_x_qdd_2ff73/1 -> Divide_ff07e/2
  Divide_ff07e/1 -> Add_e4649/1
  Divide_6b655/1 -> Add_e4649/2

== system case8/SG_D_3/d_E_fd_SG_D_3_block ==
  note: d_E_fd_SG_D_3 in case8
      | $\frac{V_{f,\mathrm{SG},D,3}-E_{\mathrm{fd},\mathrm{SG},D,3}\,K_{E}}{T_{E}}$
      | Automatically generated on 2025-10-31 19:30:15 .
  State_E_fd_SG_D_3_3a99a : Inport
  State_V_f_SG_D_3_cf6c5 : Inport  Port=2
  Add_f6aff : Sum
  Constant_-1_d5cdb : Constant  Value=-1
  Constant_K_E_f5ab2 : Constant  Value=K_E
  Constant_T_E_40aa4 : Constant  Value=T_E
  Divide_bd1b7 : Product  Inputs=*/
  Product_aaf53 : Product
  Product_e010b : Product
  Blockout_d_E_fd_SG_D_3_7634c : Outport
  wires:
  State_V_f_SG_D_3_cf6c5/1 -> Add_f6aff/2
  Constant_-1_d5cdb/1 -> Product_e010b/1
  State_E_fd_SG_D_3_3a99a/1 -> Product_e010b/2
  Constant_T_E_40aa4/1 -> Divide_bd1b7/2
  Product_e010b/1 -> Product_aaf53/1
  Product_aaf53/1 -> Add_f6aff/1
  Constant_K_E_f5ab2/1 -> Product_aaf53/2
  Divide_bd1b7/1 -> Blockout_d_E_fd_SG_D_3_7634c/1
  Add_f6aff/1 -> Divide_bd1b7/1

== system case8/SG_D_3/d_Px_1_SG_D_3_block ==
  note: d_Px_1_SG_D_3 in case8
      | $\frac{w_{\mathrm{SG},D,3}-2\,\pi \,f_{0}}{T_{w}}-\frac{\mathrm{Px}_{1,\mathrm{SG},D,3}}{T_{w}}$
      | Automatically generated on 2025-10-31 19:30:16 .
  State_Px_1_SG_D_3_05451 : Inport
  State_w_SG_D_3_d97b7 : Inport  Port=2
  Add_7cc78 : Sum
  Add_9a9f5 : Sum
  Constant_-1_3d8e3 : Constant  Value=-1
  Constant_-2.0_d94cf : Constant  Value=-2.0
  Constant_T_w_a7ad5 : Constant  Value=T_w
  Constant_T_w_f5ba9 : Constant  Value=T_w
  Constant_f0_16950 : Constant  Value=f0
  Constant_pi_c1596 : Constant  Value=pi
  Divide_b5f42 : Product  Inputs=*/
  Divide_eaf1d : Product  Inputs=*/
  Product_2597d : Product
  Product_2fb40 : Product
  Product_52183 : Product
  Blockout_d_Px_1_SG_D_3_077a4 : Outport
  wires:
  Constant_f0_16950/1 -> Product_2597d/2
  Constant_-1_3d8e3/1 -> Product_2fb40/1
  Constant_-2.0_d94cf/1 -> Product_52183/1
  Constant_pi_c1596/1 -> Product_52183/2
  Product_52183/1 -> Product_2597d/1
  State_w_SG_D_3_d97b7/1 -> Add_7cc78/2
  Divide_eaf1d/1 -> Add_9a9f5/1
  State_Px_1_SG_D_3_05451/1 -> Product_2fb40/2
  Product_2597d/1 -> Add_7cc78/1
  Product_2fb40/1 -> Divide_eaf1d/1
  Constant_T_w_a7ad5/1 -> Divide_eaf1d/2
  Add_7cc78/1 -> Divide_b5f42/1
  Constant_T_w_f5ba9/1 -> Divide_b5f42/2
  Divide_b5f42/1 -> Add_9a9f5/2
  Add_9a9f5/1 -> Blockout_d_Px_1_SG_D_3_077a4/1

== system case8/SG_D_3/d_Px_2_SG_D_3_block ==
  note: d_Px_2_SG_D_3 in case8
      | $\frac{\mathrm{Px}_{1,\mathrm{SG},D,3}-T_{2}\,\left(\frac{\mathrm{Px}_{1,\mathrm{SG},D,3}}{T_{w}}-\frac{w_{\mathrm{SG},D,3}-2\,\pi \,f_{0}}{T_{w}}\right)}{T_{1}}-\frac{\mathrm{Px}_{2,\mathrm{SG},D,3}}{T_{1}}$
      | Automatically generated on 2025-10-31 19:30:16 .
  State_Px_2_SG_D_3_6d3a4 : Inport
  State_Px_1_SG_D_3_29485 : Inport  Port=2
  State_Px_1_SG_D_3_7b549 : Inport  Port=3
  State_w_SG_D_3_f6faf : Inport  Port=4
  Add_079d4 : Sum
  Add_3c396 : Sum
  Add_d0f8a : Sum
  Add_ecbf7 : Sum
  Constant_-1_74888 : Constant  Value=-1
  Constant_-1_eae3d : Constant  Value=-1
  Constant_-2.0_dfedd : Constant  Value=-2.0
  Constant_T_1_5c1d0 : Constant  Value=T_1
  Constant_T_1_9ae13 : Constant  Value=T_1
  Constant_T_2_a8603 : Constant  Value=T_2
  Constant_T_w_01299 : Constant  Value=T_w
  Constant_T_w_7af92 : Constant  Value=T_w
  Constant_f0_5e883 : Constant  Value=f0
  Constant_pi_0c2f3 : Constant  Value=pi
  Divide_0e7b0 : Product  Inputs=*/
  Divide_2c4e8 : Product  Inputs=*/
  Divide_93f8c : Product  Inputs=*/
  Divide_ba1d9 : Product  Inputs=*/
  Product_40dcc : Product
  Product_5fe93 : Product
  Product_9121a : Product
  Product_9b9be : Product
  Product_bce64 : Product
  Blockout_d_Px_2_SG_D_3_2ce39 : Outport
  wires:
  State_Px_1_SG_D_3_7b549/1 -> Product_9121a/2
  Constant_-2.0_dfedd/1 -> Product_40dcc/1
  Constant_f0_5e883/1 -> Product_5fe93/2
  Constant_pi_0c2f3/1 -> Product_40dcc/2
  Product_40dcc/1 -> Product_5fe93/1
  State_w_SG_D_3_f6faf/1 -> Add_ecbf7/2
  Constant_-1_74888/1 -> Product_9121a/1
  Product_5fe93/1 -> Add_ecbf7/1
  Product_9121a/1 -> Divide_ba1d9/1
  Constant_T_w_7af92/1 -> Divide_ba1d9/2
  Add_ecbf7/1 -> Divide_2c4e8/1
  Constant_T_w_01299/1 -> Divide_2c4e8/2
  Divide_ba1d9/1 -> Add_079d4/1
  Divide_2c4e8/1 -> Add_079d4/2
  Constant_T_2_a8603/1 -> Product_9b9be/1
  Add_079d4/1 -> Product_9b9be/2
  Constant_-1_eae3d/1 -> Product_bce64/1
  Product_9b9be/1 -> Add_d0f8a/2
  State_Px_2_SG_D_3_6d3a4/1 -> Product_bce64/2
  State_Px_1_SG_D_3_29485/1 -> Add_d0f8a/1
  Product_bce64/1 -> Divide_0e7b0/1
  Add_3c396/1 -> Blockout_d_Px_2_SG_D_3_2ce39/1
  Constant_T_1_9ae13/1 -> Divide_0e7b0/2
  Add_d0f8a/1 -> Divide_93f8c/1
  Constant_T_1_5c1d0/1 -> Divide_93f8c/2
  Divide_0e7b0/1 -> Add_3c396/1
  Divide_93f8c/1 -> Add_3c396/2

== system case8/SG_D_3/d_Px_3_SG_D_3_block ==
  note: d_Px_3_SG_D_3 in case8
      | $\frac{\mathrm{Px}_{2,\mathrm{SG},D,3}+T_{4}\,\left(\frac{\mathrm{Px}_{1,\mathrm{SG},D,3}-T_{2}\,\left(\frac{\mathrm{Px}_{1,\mathrm{SG},D,3}}{T_{w}}-\frac{w_{\mathrm{SG},D,3}-2\,\pi \,f_{0}}{T_{w}}\right)}{T_{1}}-\frac{\mathrm{Px}_{2,\mathrm{SG},D,3}}{T_{1}}\right)}{T_{3}}-\frac{\mathrm{Px}_{3,\mathrm{SG},D,3}}{T_{3}}$
      | Automatically generated on 2025-10-31 19:30:17 .
  State_Px_3_SG_D_3_01303 : Inport
  State_Px_2_SG_D_3_61442 : Inport  Port=2
  State_Px_2_SG_D_3_31d74 : Inport  Port=3
  State_Px_1_SG_D_3_e800f : Inport  Port=4
  State_Px_1_SG_D_3_b0515 : Inport  Port=5
  State_w_SG_D_3_68c48 : Inport  Port=6
  Add_32890 : Sum
  Add_37342 : Sum
  Add_66a23 : Sum
  Add_6f360 : Sum
  Add_bdc41 : Sum
  Add_e6bb6 : Sum
  Constant_-1_43c03 : Constant  Value=-1
  Constant_-1_a7665 : Constant  Value=-1
  Constant_-1_e2890 : Constant  Value=-1
  Constant_-2.0_74c3f : Constant  Value=-2.0
  Constant_T_1_658e0 : Constant  Value=T_1
  Constant_T_1_f7794 : Constant  Value=T_1
  Constant_T_2_4629f : Constant  Value=T_2
  Constant_T_3_05bbd : Constant  Value=T_3
  Constant_T_3_d322f : Constant  Value=T_3
  Constant_T_4_f134c : Constant  Value=T_4
  Constant_T_w_3d9d0 : Constant  Value=T_w
  Constant_T_w_a9ac9 : Constant  Value=T_w
  Constant_f0_31951 : Constant  Value=f0
  Constant_pi_dc000 : Constant  Value=pi
  Divide_215df : Product  Inputs=*/
  Divide_34e1e : Product  Inputs=*/
  Divide_695b0 : Product  Inputs=*/
  Divide_97a97 : Product  Inputs=*/
  Divide_a0c46 : Product  Inputs=*/
  Divide_c0147 : Product  Inputs=*/
  Product_0413a : Product
  Product_34495 : Product
  Product_387a6 : Product
  Product_597e0 : Product
  Product_7e7fc : Product
  Product_a551b : Product
  Product_c798b : Product
  Blockout_d_Px_3_SG_D_3_3c603 : Outport
  wires:
  State_Px_1_SG_D_3_b0515/1 -> Product_34495/2
  Constant_f0_31951/1 -> Product_0413a/2
  Constant_-2.0_74c3f/1 -> Product_7e7fc/1
  Add_6f360/1 -> Divide_c0147/1
  Constant_pi_dc000/1 -> Product_7e7fc/2
  Product_7e7fc/1 -> Product_0413a/1
  State_w_SG_D_3_68c48/1 -> Add_37342/2
  Constant_T_w_a9ac9/1 -> Divide_695b0/2
  Constant_-1_e2890/1 -> Product_34495/1
  Product_0413a/1 -> Add_37342/1
  Product_34495/1 -> Divide_695b0/1
  Add_37342/1 -> Divide_215df/1
  Product_387a6/1 -> Divide_a0c46/1
  Constant_T_w_3d9d0/1 -> Divide_215df/2
  Divide_695b0/1 -> Add_e6bb6/1
  Divide_215df/1 -> Add_e6bb6/2
  Constant_T_2_4629f/1 -> Product_597e0/1
  Add_e6bb6/1 -> Product_597e0/2
  Constant_-1_43c03/1 -> Product_387a6/1
  State_Px_2_SG_D_3_31d74/1 -> Product_387a6/2
  State_Px_1_SG_D_3_e800f/1 -> Add_6f360/1
  Constant_T_3_d322f/1 -> Divide_97a97/2
  Product_597e0/1 -> Add_6f360/2
  Constant_T_1_658e0/1 -> Divide_a0c46/2
  Add_32890/1 -> Product_a551b/2
  Constant_T_1_f7794/1 -> Divide_c0147/2
  Divide_34e1e/1 -> Add_66a23/2
  Divide_a0c46/1 -> Add_32890/1
  Divide_c0147/1 -> Add_32890/2
  Constant_T_4_f134c/1 -> Product_a551b/1
  Constant_-1_a7665/1 -> Product_c798b/1
  State_Px_3_SG_D_3_01303/1 -> Product_c798b/2
  State_Px_2_SG_D_3_61442/1 -> Add_bdc41/1
  Product_a551b/1 -> Add_bdc41/2
  Product_c798b/1 -> Divide_97a97/1
  Add_bdc41/1 -> Divide_34e1e/1
  Constant_T_3_05bbd/1 -> Divide_34e1e/2
  Divide_97a97/1 -> Add_66a23/1
  Add_66a23/1 -> Blockout_d_Px_3_SG_D_3_3c603/1
